simulink model "MPPT"  (R2023b)
settings: Solver=VariableStepAuto  StartTime=0.0  StopTime=150  RelTol=1e-3
values from neighbouring files (symbols this model uses):
  Ki = 0.0011    [EI.m]
  Ti = 0.8    [EI.m]
undefined symbols (not defined in the file or in its folder): x
settings Model: Creator=padev  LastModifiedBy=33783

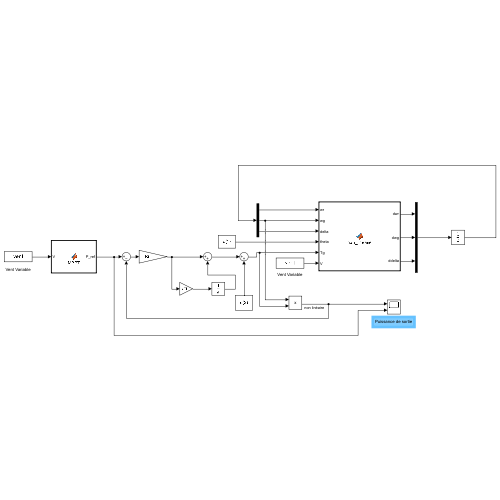
[thumbnail: Simulink's stored preview of the top-level diagram]
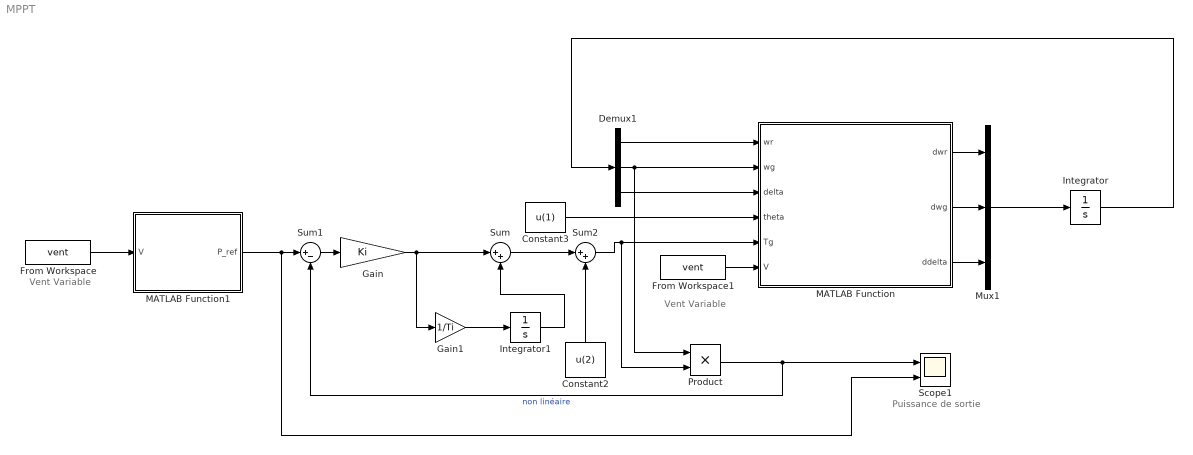
== system MPPT ==
  note: Vent Variable
  note: Puissance de sortie
  note: Vent Variable
  Constant2 : Constant  Value=u(2)
  Constant3 : Constant  Value=u(1)
  Demux1 : Demux  Outputs=3
  From Workspace : FromWorkspace  VariableName=vent
  From Workspace1 : FromWorkspace  VariableName=vent
  Gain : Gain  Gain=Ki
  Gain1 : Gain  Gain=1/Ti
  Integrator : Integrator  InitialCondition=[x(1),x(2),x(3)]
  Integrator1 : Integrator
  MATLAB Function : MATLAB Function  TreatAsAtomicUnit=on
  MATLAB Function1 : MATLAB Function  TreatAsAtomicUnit=on
  Mux1 : Mux  Inputs=3
  Product : Product
  Scope1 : Scope  NumInputPorts=2
  Sum : Sum  Inputs=|++
  Sum1 : Sum  Inputs=|+-
  Sum2 : Sum  Inputs=|++
  wires:
  Demux1/3 -> MATLAB Function/3(delta)
  MATLAB Function/1(dwr) -> Mux1/1
  Mux1/1 -> Integrator/1
  Demux1/2 -> Product/1, MATLAB Function/2(wg)
  Demux1/1 -> MATLAB Function/1(wr)
  Constant3/1 -> MATLAB Function/4(theta)
  MATLAB Function/3(ddelta) -> Mux1/3
  Integrator/1 -> Demux1/1
  MATLAB Function/2(dwg) -> Mux1/2
  Product/1 -> Scope1/1, Sum1/2  "non linéaire"
  Gain/1 -> Sum/1, Gain1/1
  Sum1/1 -> Gain/1
  Gain1/1 -> Integrator1/1
  Integrator1/1 -> Sum/2
  Sum/1 -> Sum2/1
  Sum2/1 -> Product/2, MATLAB Function/5(Tg)
  Constant2/1 -> Sum2/2
  MATLAB Function1/1(P_ref) -> Scope1/2, Sum1/1
  From Workspace/1 -> MATLAB Function1/1(V)
  From Workspace1/1 -> MATLAB Function/6(V)

== matlab function MPPT/MATLAB Function1 ==
  data: P_ref output; V input
function P_ref  = MPPT(V)
    %% Représentation d'état non linéaire :
    % Valeurs du modèle :
    R = 21.65 ; % en mètres
    rho = 1.292 ; % en kg/m3
  
    P_ref = 0.5*rho*pi*(R^2)*(V^3)*0.347;

== matlab function MPPT/MATLAB Function ==
  data: wr input; dwr output; wg input; delta input; theta input; Tg input; dwg output; ddelta output; V input
function [dwr,dwg,ddelta] = non_lineaire(wr,wg,delta,theta,Tg,V)
    %% Représentation d'état non linéaire :
    % Valeurs du modèle :
    n_g = 43.165 ; % sans unité
    J_r = 3.25e5 ; % kg/m^2
    J_g = 34.4 ; % kg/m^2
    K_s = 269.1e3 ; % N.m/rad
    R = 21.65 ; % en mètres
    rho = 1.292 ; % en kg/m3
  
    D_s= 9500; % Nm/rad/s
    
   
    function Lambdai = funLambdai(lambda,theta)
        Lambdai = 1/(1/(lambda+0.08*theta)- 0.035/(theta^3 + 1)) ;
    end
    
    function Cp = funCp(lambda,theta) 
        Cp = 0.5*(116/funLambdai(lambda,theta)-0.4*theta-5)*exp(-21/funLambdai(lambda,theta)) + 0.0068*lambda ;
    end
    
    % Puissance 
    function Pr = funPuissance(wr,theta,V)
        lambda=(wr*R)/V;
        Pr = 0.5*rho*pi*(R^2)*(V^3)*funCp(lambda,theta);
    end
    
    dwr = 1/(J_r*wr) * funPuissance(wr,theta,V) - (D_s/J_r) * wr + (D_s/(J_r*n_g)) * wg - (K_s/J_r) * delta ;
    dwg = (D_s/(J_g * n_g)) * wr - (D_s/(J_g * n_g^2)) * wg + (K_s/(J_g * n_g)) * delta - (1/J_g) * Tg ;
    ddelta = wr - 1/n_g * wg;

    end
